simulink model "interp_1"  (Simulink 7.8)
settings: Solver=ode45  StartTime=0.0  StopTime=1  RelTol=1e-3
undefined symbols (not defined in the file or in its folder): get, One, sided
libraries: dspsigops x3, dsparch4 x1, dspsnks4 x1
settings Model: Creator=svenhoffmann  LastModifiedBy=josef  ExtModeAutoUpdateStatusClock=off
settings DataIOCC: SignalLoggingName=sigsOut
settings OptimizationCC: InitFltsAndDblsToZero=on
settings DebuggingCC: SaveWithParameterizedLinksMsg=none  SignalResolutionControl=TryResolveAllWithWarning  SolverPrmCheckMsg=none  MultiTaskDSMMsg=warning  MultiTaskCondExecSysMsg=none  FcnCallInpInsideContextMsg=Use local settings  StrictBusMsg=None
settings HardwareCC: TargetUnknown=on
settings RTWCC: IncludeERTFirstTime=on
settings GRTTargetCC: TargetFcnLib=ansi_tfl_tmw.mat

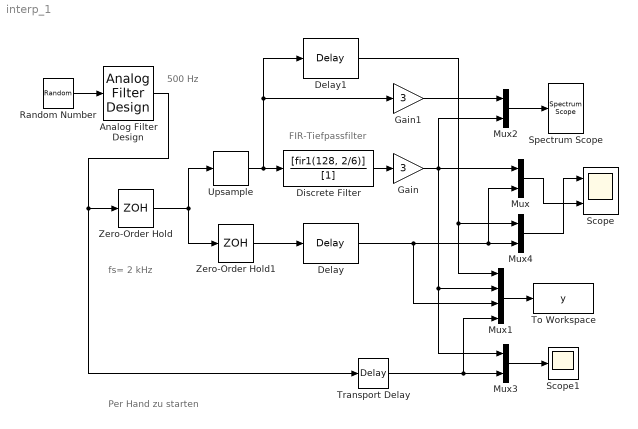
== system interp_1 ==
  note: 500 Hz
  note: fs=
      | 2 kHz
  note: FIR-Tiefpassfilter
  note: Per Hand zu starten
  Analog Filter Design : dsparch4/Analog Filter Design  method=Elliptic  filttype=Lowpass  N=8  Wlo=2*pi*600  Whi=80  Rp=2  Rs=40
  Delay : dspsigops/Delay  InputProcessing=Inherited (this choice will be removed - see release notes)  dly_unit=Samples  delay=64  ic_detail=off  dif_ic_for_ch=off  dif_ic_for_dly=off  ic=0  reset_popup=None
  Delay1 : dspsigops/Delay  InputProcessing=Inherited (this choice will be removed - see release notes)  dly_unit=Samples  delay=64  ic_detail=off  dif_ic_for_ch=off  dif_ic_for_dly=off  ic=0  reset_popup=None
  Discrete Filter : DiscreteFilter  Numerator=[fir1(128, 2/6)]  Denominator=[1]  SampleTime=1/6000
  Gain : Gain  Gain=3  SaturateOnIntegerOverflow=on  OutDataTypeStr=Inherit: Same as input  ParamDataTypeStr=Inherit: Same as input
  Gain1 : Gain  Gain=3  SaturateOnIntegerOverflow=on  OutDataTypeStr=Inherit: Same as input  ParamDataTypeStr=Inherit: Same as input
  Mux{,2..4} (4 alike) : Mux  Inputs=2
  Mux1 : Mux
  Random Number : RandomNumber  SampleTime=0
  Scope : Scope  NumInputPorts=2
      settings: TimeRange=0.009929971988795519  YMin=-1.2~-1.92568  YMax=1.1~1.4527
  Scope1 : Scope
  Spectrum Scope : dspsnks4/Spectrum Scope  ScopeProperties=on  Domain=Frequency  HorizSpan=1  UseBuffer=on  BufferSize=256  Overlap=64  TreatMby1Signals=M channels  inpFftLenInherit=off  FFTlength=128  numAvg=10  DisplayProperties=off  AxisGrid=on  Memory=off  FrameNumber=on  AxisLegend=off  AxisZoom=off  OpenScopeAtSimStart=on  OpenScopeImmediately=off  FigPos=get(0,'defaultfigureposition')  AxisProperties=off  XUnits=Hertz  XRange=One-sided ([0...Fs/2])  XDisplay=0  InheritXIncr=off  XIncr=1/6000  XLabel=Samples  XLimit=Auto  YUnits=dBW/Hertz  XMax=1  XMin=0  YLabel=Magnitude, dB  LineProperties=off  wintypeSpecScope=Hann  RsSpecScope=50  betaSpecScope=5  winsampSpecScope=Periodic  XAxisParamsVer=6.8  isFrameUpgraded=on
      settings: YMin=-151.9779  YMax=-35.6173
  To Workspace : ToWorkspace  VariableName=y  SampleTime=-1  SaveFormat=Structure With Time
  Transport Delay : TransportDelay  DelayTime=64/6000
  Upsample : dspsigops/Upsample  N=3  phase=0  InputProcessing=Inherited (this choice will be removed - see release notes)  RateOptions=Allow multirate processing  ic=0  mode=Unused parameter value
  Zero-Order Hold : ZeroOrderHold  SampleTime=1/2000
  Zero-Order Hold1 : ZeroOrderHold  SampleTime=1/6000
  wires:
  Zero-Order Hold/1 -> Upsample/1, Zero-Order Hold1/1
  Discrete Filter/1 -> Gain/1
  Mux1/1 -> To Workspace/1
  Mux2/1 -> Spectrum Scope/1
  Upsample/1 -> Discrete Filter/1, Gain1/1, Delay1/1
  Gain/1 -> Mux2/2, Mux/1, Mux1/2, Mux3/1
  Delay/1 -> Mux1/3, Mux/2, Mux4/2
  Zero-Order Hold1/1 -> Delay/1
  Random Number/1 -> Analog Filter Design/1
  Analog Filter Design/1 -> Zero-Order Hold/1, Transport Delay/1
  Mux3/1 -> Scope1/1
  Transport Delay/1 -> Mux3/2, Mux1/4
  Gain1/1 -> Mux2/1
  Delay1/1 -> Mux1/1, Mux4/1
  Mux/1 -> Scope/2
  Mux4/1 -> Scope/1
